simulink model "Counter"  (Simulink 8.4)
settings: Solver=FixedStepDiscrete  StartTime=0.0  StopTime=20.0  FixedStep=1.0  RelTol=1e-3
settings Model: Creator=arnaud  LastModifiedBy=arnaud

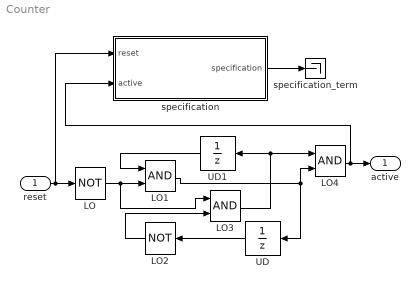
== system Counter ==
  reset : Inport  OutDataTypeStr=boolean
  LO : Logic  Operator=NOT  AllPortsSameDT=off  OutDataTypeStr=boolean
  LO1 : Logic  AllPortsSameDT=off  OutDataTypeStr=boolean
  LO2 : Logic  Operator=NOT  AllPortsSameDT=off  OutDataTypeStr=boolean
  LO3 : Logic  AllPortsSameDT=off  OutDataTypeStr=boolean
  LO4 : Logic  AllPortsSameDT=off  OutDataTypeStr=boolean
  UD : UnitDelay  InitialCondition=false
  UD1 : UnitDelay  InitialCondition=false
  specification : Subsystem  TreatAsAtomicUnit=on  mask(Observer){AnnotationType=ensures, ObserverType=[]}
      mask prompts: AnnotationType "Type of annotation (pre/post...)"; ObserverType "Observer type"
      mask help:
      | Set an observer for the system.
      | The annotation type parameter sets the type of observer:
      | - requires : pre-condition
      | - ensures : post-condition
      | - assert : an assertion
      | - observer : the observer computes a special type of properties
      mask TypeOptions AnnotationType: ensures | requires | assert | observer
      mask Callback AnnotationType:
      | paramStr = get_param(gcb, 'MaskValues');
      | if strcmp(paramStr{1}(1),'o')
      | set_param(gcb,'MaskVisibilities',{'on';'on'});
      | paramStr{2} = 'ellipsoid';
      | set_param(gcb,'MaskValues',paramStr);
      | else
      | set_param(gcb,'MaskVisibilities',{'on';'off'});
      | end
      mask Callback ObserverType:
      | paramStr = get_param(gcb, 'MaskValues');
      | if strcmp(paramStr{1}(1),'o')
      | set_param(gcb,'MaskVisibilities',{'on';'on'});
      | paramStr{2} = 'ellipsoid';
      | set_param(gcb,'MaskValues',paramStr);
      | else
      | set_param(gcb,'MaskVisibilities',{'on';'off'});
      | end
      mask Display:
      | color('black')
      | text(0.5, 0.5, ['Property: ''' get_param(gcb,'name') ''''], 'horizontalAlignment', 'center');
      | text(0.99, 0.03, '{\bf\fontsize{12}SAFE}', 'hor', 'right', 'ver', 'bottom', 'texmode', 'on');
  specification_term : Terminator
  active : Outport
  wires:
  reset/1 -> LO/1, specification/1(reset)
  LO/1 -> LO1/2, LO3/1
  UD/1 -> LO2/1
  LO2/1 -> LO3/2
  UD1/1 -> LO1/1
  LO1/1 -> UD/1, LO4/2
  LO3/1 -> UD1/1, LO4/1
  LO4/1 -> active/1, specification/2(active)
  specification/1(specification) -> specification_term/1

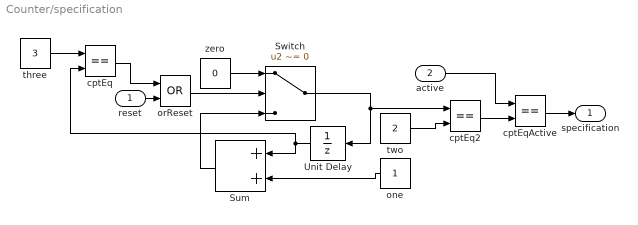
== system Counter/specification ==
  reset : Inport
  active : Inport  Port=2
  Sum : Sum
  Switch : Switch  Criteria=u2 ~= 0
  Unit Delay : UnitDelay
  cptEq : RelationalOperator  Operator===  OutDataTypeStr=boolean
  cptEq2 : RelationalOperator  Operator===  OutDataTypeStr=boolean
  cptEqActive : RelationalOperator  Operator===  OutDataTypeStr=boolean
  one : Constant
  orReset : Logic  Operator=OR  AllPortsSameDT=off  OutDataTypeStr=boolean
  three : Constant  Value=3
  two : Constant  Value=2
  zero : Constant  Value=0
  specification : Outport
  wires:
  zero/1 -> Switch/1
  two/1 -> cptEq2/2
  cptEq2/1 -> cptEqActive/2
  active/1 -> cptEqActive/1
  reset/1 -> orReset/2
  cptEq/1 -> orReset/1
  orReset/1 -> Switch/2
  Switch/1 -> Unit Delay/1, cptEq2/1
  Unit Delay/1 -> Sum/1, cptEq/2
  one/1 -> Sum/2
  Sum/1 -> Switch/3
  three/1 -> cptEq/1
  cptEqActive/1 -> specification/1
